simulink model "ModelMedusa"  (R2022b)
settings: Solver=FixedStepDiscrete  StartTime=0.0  StopTime=1  RelTol=1e-3  EnableMultiTasking=on
InitFcn:
  | % Initialize model
  | run(['ModelInit.m']);
  | 
  | % load library data
  | GainLibrary_data;
StartFcn:
  | % make sure all the simulated RTC requests are found
  | %RTC_SIM_OBJ.ValidateREQs();
model workspace (MAT data in the model file):
  PreampVolumeTable_Idx = Simulink.Signal
  PreampVolumeTable_Idx.DataType = 'auto'
  PreampVolumeTable_Idx.Dimensions = -1
  PreampVolumeTable_Idx.DimensionsMode = 'auto'
  PreampVolumeTable_Idx.Complexity = 'auto'
  PreampVolumeTable_Idx.SampleTime = -1
  PreampVolumeTable_Idx.SamplingMode = 'auto'
  PreampVolumeTable_Idx.InitialValue = 'uint8([0 255 255 255 255 255])'
  Range = Simulink.Signal
  Range.DataType = 'auto'
  Range.Dimensions = -1
  Range.DimensionsMode = 'auto'
  Range.Complexity = 'auto'
  Range.SampleTime = -1
  Range.SamplingMode = 'auto'
  Table_Idx = Simulink.Signal
  Table_Idx.DataType = 'auto'
  Table_Idx.Dimensions = -1
  Table_Idx.DimensionsMode = 'auto'
  Table_Idx.Complexity = 'auto'
  Table_Idx.SampleTime = -1
  Table_Idx.SamplingMode = 'auto'
undefined symbols (not defined in the file): Config, IFIR, Ifir, MedusaConfig, numAudioIn, Row, sys_defs, VLSConfig
libraries: TuneVar x16, FeaturePath x15, MedusaDelays x9, RTC x5, TOP x5, SampleRateConverter x4, dspindex x3, EdgePorts x2, MedusaCaeEnable x2, FIREven x2, VLSGains x2, dspsrcs4 x2
(part 1 of 2)
settings Model: Creator=kl13806  LastModifiedBy=sc48041
settings SolverCC: AlgebraicLoopSolver=TrustRegion  AutoInsertRateTranBlk=on
settings OptimizationCC: DefaultParameterBehavior=Inlined  DefaultUnderspecifiedDataType=single  ZeroExternalMemoryAtStartup=off  ZeroInternalMemoryAtStartup=off  MaxStackSize=2048  DifferentSizesBufferReuse=on  EfficientTunableParamExpr=on
settings DebuggingCC: InheritedTsInSrcMsg=none  MultiTaskDSMMsg=none  MultiTaskRateTransMsg=warning  ParameterPrecisionLossMsg=none  ParameterTunabilityLossMsg=error  UnconnectedInputMsg=warning  UnconnectedOutputMsg=warning  UnconnectedLineMsg=warning  BusObjectLabelMismatch=none  UnknownTsInhSupMsg=none  SFUnexpectedBacktrackingDiag=warning  SFNoUnconditionalDefaultTransitionDiag=warning  SFExecutionAtInitializationDiag=none  SFMachineParentedDataDiag=warning  ArithmeticOperatorsInVariantConditions=warning
settings HardwareCC: ProdBitPerDouble=32  ProdBitPerPointer=32  ProdBitPerSizeT=32  ProdBitPerPtrDiffT=32  ProdLargestAtomicInteger=Long  ProdLargestAtomicFloat=Double  ProdWordSize=32  ProdHWDeviceType=Qualcomm->Hexagon  TargetBitPerPointer=64  TargetBitPerSizeT=64  TargetBitPerPtrDiffT=64  TargetLargestAtomicInteger=Integer  TargetLongLongMode=on  TargetIntDivRoundTo=Zero  TargetEndianess=LittleEndian  TargetWordSize=64  TargetHWDeviceType=MATLAB Host  ProdEqTarget=off
settings ModelReferenceCC: EnableRefExpFcnMdlSchedulingChecks=on
settings SFSimCC: SimUseLocalCustomCode=off  MATLABDynamicMemAlloc=off  CustomCodeUndefinedFunction=UseInterfaceOnly
settings RTWCC: Description=Embedded Coder (host-based shared library target)  SystemTargetFile=ert_shrlib.tlc  GenCodeOnly=on  TemplateMakefile=ert_default_tmf  GenerateReport=on  RetainRTWFile=on  RTWUseLocalCustomCode=off  BuildConfiguration=Faster Runs  IncludeHyperlinkInReport=on  LaunchReport=on  GenerateTraceInfo=on  GenerateTraceReport=on  GenerateTraceReportSl=on  GenerateTraceReportSf=on  GenerateTraceReportEml=on  GenerateCodeMetricsReport=on  GenerateCodeReplacementReport=on
settings CodeAppCC: ForceParamTrailComments=on  IgnoreCustomStorageClasses=off  MaxIdLength=61  OperatorAnnotations=on  SimulinkDataObjDesc=on  SFDataObjDesc=on  MATLABFcnDesc=on  InsertBlockDesc=on  StateflowObjectComments=on  MATLABSourceComments=on
settings STFCustomTargetCC: TargetLangStandard=C99 (ISO)  CodeReplacementLibrary=Qualcomm Hexagon DSP code replacement library  ParMdlRefBuildCompliant=on  CompOptLevelCompliant=on  CombineOutputUpdateFcns=on  ERTCustomFileBanners=on  SupportNonFinite=off  SupportContinuousTime=off  SupportNonInlinedSFcns=off  RemoveResetFunc=on  SupportVariableSizeSignals=on  MATLABClassNameForMDSCustomization=Simulink.SoftwareTarget.ERTCustomization  ModelStepFunctionPrototypeControlCompliant=on  UseToolchainInfoCompliant=on  SystemTargetFile=ert_shrlib.tlc
settings ERTTargetCC: TargetLangStandard=C99 (ISO)  CodeReplacementLibrary=Qualcomm Hexagon DSP code replacement library  MultiwordLength=2048  ConcurrentExecutionCompliant=off  SupportNonFinite=off  SupportVariableSizeSignals=on  CPPClassGenCompliant=off  InlinedParameterPlacement=NonHierarchical  ERTCustomFileTemplate=example_file_process.tlc  IndentStyle=Allman  IndentSize=4
settings ConfigComp: CovMetricSettings=dw  CovSaveCumulativeToWorkspaceVar=on  CovSaveSingleToWorkspaceVar=on  CovExternalEMLEnable=off

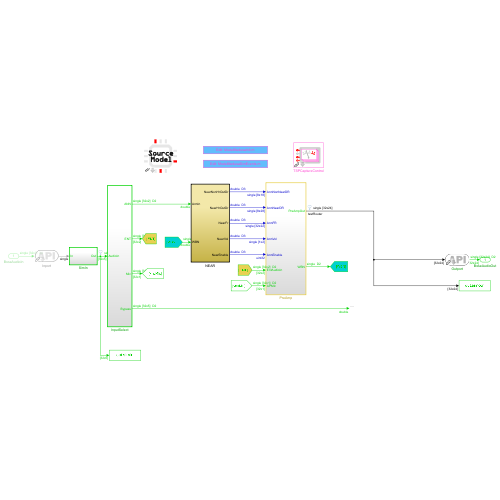
[thumbnail: Simulink's stored preview of the top-level diagram]
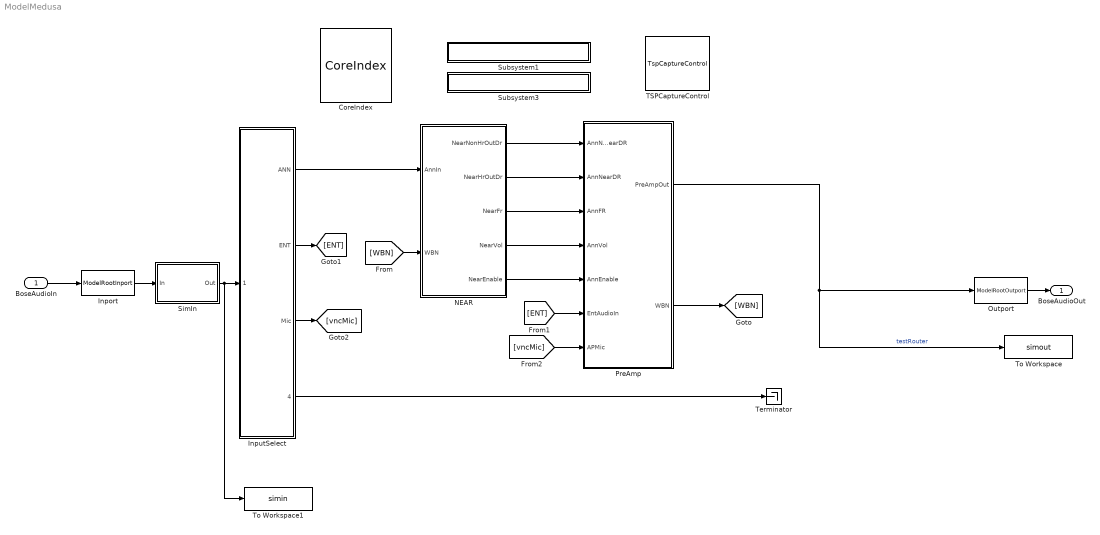
== system ModelMedusa ==
  BoseAudioIn : Inport  OutDataTypeStr=single  PortDimensions=[sys_defs.frameSize numAudioIn]  SampleTime=1/sys_defs.Fs * sys_defs.frameSize
  CoreIndex : FeaturePath/CoreIndex  Role=Source Model  CoreIndex=8  Config=[]  AddressingMode=Directly include core number in message identifiers (i.e. simple and static)  CrossCoreApi=None  CrossCoreAllocation=None  CrossCoreSampleTime=-1  BasePeriod=[]  TriggerInit=[-15 -776 80 -679]
      settings: SourceProductName=Bose Talaria
  Inport : EdgePorts/ModelRootInport  Config=ModelRootIn
      settings: SourceProductName=Bose Talaria
  InputSelect : Subsystem  TreatAsAtomicUnit=on
      settings: RTWSystemCode=Nonreusable function
  NEAR : Subsystem  TreatAsAtomicUnit=on
  Outport : EdgePorts/ModelRootOutport  Config=ModelRootOut
      settings: SourceProductName=Bose Talaria
  PreAmp : Subsystem  TreatAsAtomicUnit=on
  SimIn : Subsystem  TreatAsAtomicUnit=on
  Subsystem1 : Subsystem  mask{filename=Init.m}
      settings: OpenFcn=edit([ ModelRootName() get(gcbh,'filename') ]);
      mask Display: disp(['Edit: ' ModelRootName() get(gcbh,'filename')]);
  Subsystem3 : Subsystem  mask{filename=SimEvents.m}
      settings: OpenFcn=edit([ ModelRootName() get(gcbh,'filename') ]);
      mask Display: disp(['Edit: ' ModelRootName() get(gcbh,'filename')]);
  TSPCaptureControl : TSP/TspCaptureControl  TriggerInit=[415 -766 500 -694]
      settings: SourceProductName=Bose Talaria
  Terminator : Terminator
  To Workspace : ToWorkspace  VariableName=simout  SaveFormat=Timeseries  SampleTime=-1
  To Workspace1 : ToWorkspace  VariableName=simin  SaveFormat=Timeseries  SampleTime=-1
  BoseAudioOut : Outport  VectorParamsAs1DForOutWhenUnconnected=off
  wires:
  SimIn/1(Out) -> To Workspace1/1, InputSelect/1(AudioIn)
  BoseAudioIn/1 -> Inport/1
  Inport/1 -> SimIn/1(In)
  Outport/1 -> BoseAudioOut/1
  InputSelect/1(ANN) -> NEAR/1(AnnIn)
  [WBN] -> NEAR/2(WBN)
  NEAR/5(NearEnable) -> PreAmp/5(AnnEnable)
  NEAR/4(NearVol) -> PreAmp/4(AnnVol)
  NEAR/3(NearFr) -> PreAmp/3(AnnFR)
  PreAmp/2(WBN) -> [WBN]
  NEAR/1(NearNonHrOutDr) -> PreAmp/1(AnnNonNearDR)
  NEAR/2(NearHrOutDr) -> PreAmp/2(AnnNearDR)
  InputSelect/2(ENT) -> [ENT]
  [ENT] -> PreAmp/6(EntAudioIn)
  InputSelect/3(Mic) -> [vncMic]
  [vncMic] -> PreAmp/7(APMic)
  InputSelect/4(Bypass) -> Terminator/1
  PreAmp/1(PreAmpOut) -> To Workspace/1, Outport/1  "testRouter"

== system ModelMedusa/InputSelect ==
  AudioIn : Inport
  FeaturePath : FeaturePath/FeaturePath  FeatureName=InputSelect  IsGroup=on  GroupNumber=0  IsModule=on  TriggerInit=[105 216 220 329]
      settings: SourceProductName=Bose Talaria
  Partition : FeaturePath/Partition  PartitionNumber=0  TriggerInit=[250 241 295 309]
      settings: SourceProductName=Bose Talaria
  Reset : Subsystem  Commented=on
  Variable Selector1 : dspindex/Variable Selector  NumInputs=1  rowsOrCols=Columns  IdxMode=Fixed  Elements=entMap  ZerOneIdxMode=One-based  errmode=Clip Index  FillMode=on  FillValues=0
  Variable Selector2 : dspindex/Variable Selector  NumInputs=1  rowsOrCols=Columns  IdxMode=Fixed  Elements=annMap  ZerOneIdxMode=One-based  errmode=Clip Index  FillMode=on  FillValues=0
  Variable Selector3 : dspindex/Variable Selector  NumInputs=1  rowsOrCols=Columns  IdxMode=Fixed  Elements=vncMic  ZerOneIdxMode=One-based  errmode=Clip Index  FillMode=on  FillValues=0
  router : Router/Router  nInRouterMask=inputSelectChanIn  nOutRouterMask=inputSelectChanOut  outputMapDefaultRouterMask=inputSelectOutputMap
  ANN : Outport
  ENT : Outport  Port=2  VectorParamsAs1DForOutWhenUnconnected=off
  Mic : Outport  Port=3
  Bypass : Outport  Port=4  VectorParamsAs1DForOutWhenUnconnected=off
  wires:
  Variable Selector1/1 -> ENT/1
  AudioIn/1 -> Bypass/1, router/1
  router/1 -> Variable Selector3/1, Variable Selector2/1, Variable Selector1/1
  Variable Selector2/1 -> ANN/1
  Variable Selector3/1 -> Mic/1

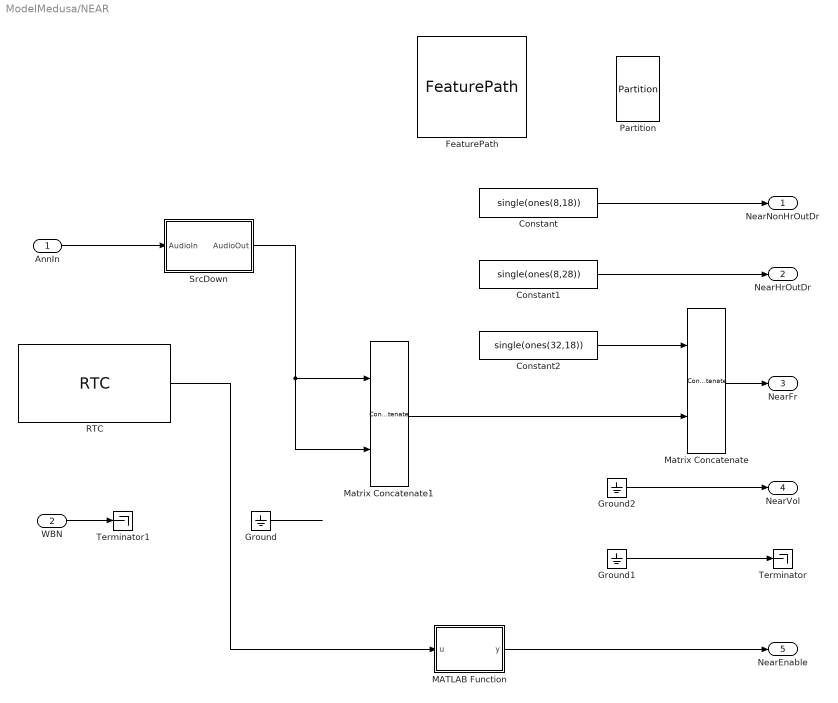
== system ModelMedusa/NEAR ==
  AnnIn : Inport
  WBN : Inport  Port=2
  Constant : Constant  Value=single(ones(8,18))
  Constant1 : Constant  Value=single(ones(8,28))
  Constant2 : Constant  Value=single(ones(32,18))
  FeaturePath : FeaturePath/FeaturePath  FeatureName=Near  IsGroup=on  GroupNumber=1  IsModule=on  TriggerInit=[15 -306 130 -199]
      settings: SourceProductName=Bose Talaria
  Ground : Ground
  Ground1 : Ground
  Ground2 : Ground
  MATLAB Function : MATLAB Function  TreatAsAtomicUnit=on
  Matrix Concatenate : Concatenate  Mode=Multidimensional array  ConcatenateDimension=2
  Matrix Concatenate1 : Concatenate  Mode=Multidimensional array  ConcatenateDimension=2
  Partition : FeaturePath/Partition  PartitionNumber=0  TriggerInit=[225 -284 270 -216]
      settings: SourceProductName=Bose Talaria
  RTC : RTC/RTC  REQ_Priority=RTC_Mask.NormalPriority  RequestAtInit=off  EnableRequest=off  REQElemName1=Enable  REQElemType1=uint32  REQElemWidth1=1  REQElemInitial1=[0]  REQElemType2=uint32  REQElemWidth2=1  REQElemInitial2=[]  REQElemType3=uint32  REQElemWidth3=1  REQElemInitial3=[]  REQElemType4=uint32  REQElemWidth4=1  REQElemInitial4=[]  REQElemType5=uint32  REQElemWidth5=1  REQElemInitial5=[]  REQElemType6=uint32  REQElemWidth6=1  REQElemInitial6=[]  REQElemType7=uint32  REQElemWidth7=1  REQElemInitial7=[]  REQElemType8=uint32  REQElemWidth8=1  REQElemInitial8=[]  REQElemType9=uint32  REQElemWidth9=1  REQElemInitial9=[]  REQElemType10=uint32  REQElemWidth10=1  REQElemInitial10=[]  EnableResponse=on  EnableRSP_StatusIn=off  RSPElemType1=uint32  RSPElemWidth1=1  RSPElemType2=uint32  RSPElemWidth2=1  RSPElemType3=uint32  RSPElemWidth3=1  RSPElemType4=uint32  RSPElemWidth4=1  RSPElemType5=uint32  RSPElemWidth5=1  RSPElemType6=uint32  RSPElemWidth6=1  RSPElemType7=uint32  RSPElemWidth7=1  RSPElemType8=uint32  RSPElemWidth8=1  RSPElemType9=uint32  RSPElemWidth9=1  RSPElemType10=uint32  RSPElemWidth10=1  EnableNotification=off  EnableNTF_PrepTrig=off  NTFElemType1=uint32  NTFElemWidth1=1  NTFElemType2=uint32  NTFElemWidth2=1  NTFElemType3=uint32  NTFElemWidth3=1  NTFElemType4=uint32  NTFElemWidth4=1  NTFElemType5=uint32  NTFElemWidth5=1  NTFElemType6=uint32  NTFElemWidth6=1  NTFElemType7=uint32  NTFElemWidth7=1  NTFElemType8=uint32  NTFElemWidth8=1  NTFElemType9=uint32  NTFElemWidth9=1  NTFElemType10=uint32  NTFElemWidth10=1  MaskMessageName=Enable
      settings: SourceProductName=Bose Talaria
  SrcDown : Subsystem  TreatAsAtomicUnit=on
      settings: RTWSystemCode=Nonreusable function
  Terminator : Terminator
  Terminator1 : Terminator
  NearNonHrOutDr : Outport
  NearHrOutDr : Outport  Port=2
  NearFr : Outport  Port=3
  NearVol : Outport  Port=4
  NearEnable : Outport  Port=5
  wires:
  Constant/1 -> NearNonHrOutDr/1
  AnnIn/1 -> SrcDown/1(AudioIn)
  Constant1/1 -> NearHrOutDr/1
  Constant2/1 -> Matrix Concatenate/1
  Matrix Concatenate1/1 -> Matrix Concatenate/2
  Matrix Concatenate/1 -> NearFr/1
  Ground2/1 -> NearVol/1
  Ground1/1 -> Terminator/1
  RTC/1 -> MATLAB Function/1(u)
  MATLAB Function/1(y) -> NearEnable/1
  SrcDown/1(AudioOut) -> Matrix Concatenate1/2, Matrix Concatenate1/1
  Ground/1 -> ?
  WBN/1 -> Terminator1/1

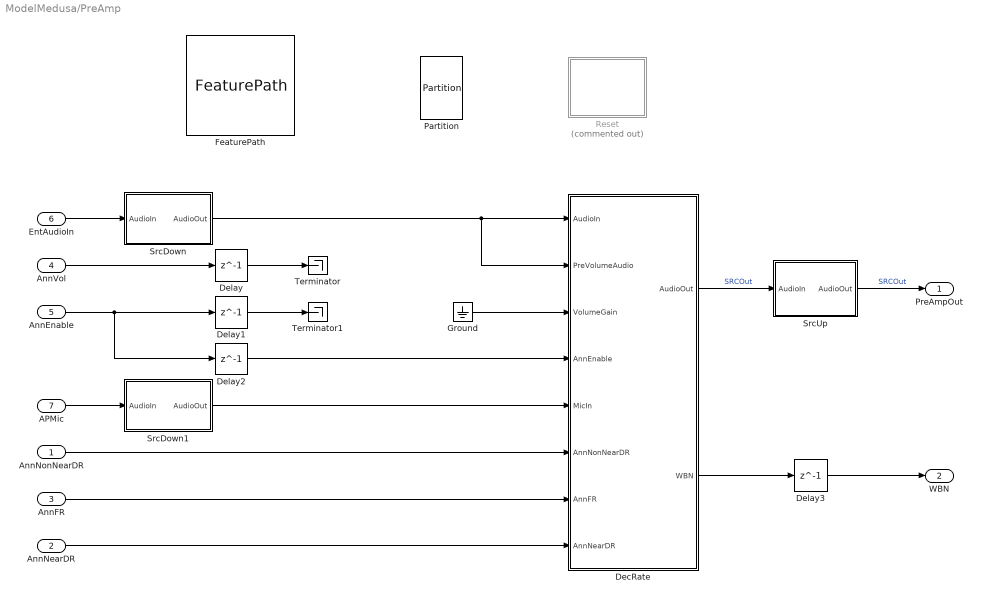
== system ModelMedusa/PreAmp ==
  AnnNonNearDR : Inport
  AnnNearDR : Inport  Port=2
  AnnFR : Inport  Port=3
  AnnVol : Inport  Port=4
  AnnEnable : Inport  Port=5
  EntAudioIn : Inport  Port=6
  APMic : Inport  Port=7
  DecRate : Subsystem
  Delay{,1..3} (4 alike) : Delay  DelayLength=1
  FeaturePath : FeaturePath/FeaturePath  FeatureName=PreAmp  IsGroup=on  GroupNumber=2  IsModule=on  TriggerInit=[-135 -246 -20 -139]
      settings: SourceProductName=Bose Talaria
  Ground : Ground
  Partition : FeaturePath/Partition  PartitionNumber=0  TriggerInit=[115 -224 160 -156]
      settings: SourceProductName=Bose Talaria
  Reset : Subsystem  Commented=on
  SrcDown : Subsystem  TreatAsAtomicUnit=on
      settings: RTWSystemCode=Nonreusable function
  SrcDown1 : Subsystem  TreatAsAtomicUnit=on
      settings: RTWSystemCode=Nonreusable function
  SrcUp : Subsystem  TreatAsAtomicUnit=on
      settings: RTWSystemCode=Nonreusable function
  Terminator : Terminator
  Terminator1 : Terminator
  PreAmpOut : Outport  VectorParamsAs1DForOutWhenUnconnected=off
  WBN : Outport  Port=2
  wires:
  EntAudioIn/1 -> SrcDown/1(AudioIn)
  DecRate/1(AudioOut) -> SrcUp/1(AudioIn)  "SRCOut"
  SrcUp/1(AudioOut) -> PreAmpOut/1  "SRCOut"
  Delay3/1 -> WBN/1
  AnnVol/1 -> Delay/1
  AnnEnable/1 -> Delay2/1, Delay1/1
  Delay/1 -> Terminator/1
  Delay1/1 -> Terminator1/1
  AnnNonNearDR/1 -> DecRate/6(AnnNonNearDR)
  AnnNearDR/1 -> DecRate/8(AnnNearDR)
  AnnFR/1 -> DecRate/7(AnnFR)
  APMic/1 -> SrcDown1/1(AudioIn)
  SrcDown/1(AudioOut) -> DecRate/2(PreVolumeAudio), DecRate/1(AudioIn)
  Ground/1 -> DecRate/3(VolumeGain)
  Delay2/1 -> DecRate/4(AnnEnable)
  DecRate/2(WBN) -> Delay3/1
  SrcDown1/1(AudioOut) -> DecRate/5(MicIn)

== system ModelMedusa/SimIn ==
  In : Inport  OutDataTypeStr=single  SampleTime=1/sys_defs.Fs * sys_defs.frameSize
  Colored Noise : dspsrcs4/Colored Noise  Commented=on  Color=pink  InverseFrequencyPower=1  BoundedOutput=on  NumChannels=2  OutputDataType=single  SamplesPerFrame=32  SampleTime=1/48000  RandomStream=mt19937ar with seed  Seed=67  SimulateUsing=Interpreted execution
  Sine Wave : dspsrcs4/Sine Wave  Amplitude=[0.1*ones(1,numAudioIn)]  Frequency=[150 225 200 275 325]  Phase=zeros(1,numAudioIn)  SampleMode=Discrete  OutComplex=Real  CompMethod=Trigonometric fcn  TableSize=Speed  SampleTime=1/sys_defs.Fs  SamplesPerFrame=sys_defs.frameSize  ResetState=Restart at time zero  OutputFrames=off  dataType=single  wordLen=16  udDataType=sfix(16)  fracBitsMode=Best precision  numFracBits=15  OutDataTypeStr=single  LastOutDataTypeStr=single
  Variant Source : VariantSource  VariantControlMode=sim codegen switching  ShowConditionOnBlock=on
  Out : Outport  VectorParamsAs1DForOutWhenUnconnected=off
  wires:
  In/1 -> Variant Source/2
  Variant Source/1 -> Out/1
  Sine Wave/1 -> Variant Source/1

== system ModelMedusa/Subsystem1 ==

== system ModelMedusa/Subsystem3 ==

== system ModelMedusa/InputSelect/Reset ==
  MATLAB Function : MATLAB Function  TreatAsAtomicUnit=on
  RTC : RTC/RTC  REQ_Priority=RTC_Mask.NormalPriority  RequestAtInit=off  EnableRequest=on  REQElemType1=uint32  REQElemWidth1=1  REQElemInitial1=[]  REQElemType2=uint32  REQElemWidth2=1  REQElemInitial2=[]  REQElemType3=uint32  REQElemWidth3=1  REQElemInitial3=[]  REQElemType4=uint32  REQElemWidth4=1  REQElemInitial4=[]  REQElemType5=uint32  REQElemWidth5=1  REQElemInitial5=[]  REQElemType6=uint32  REQElemWidth6=1  REQElemInitial6=[]  REQElemType7=uint32  REQElemWidth7=1  REQElemInitial7=[]  REQElemType8=uint32  REQElemWidth8=1  REQElemInitial8=[]  REQElemType9=uint32  REQElemWidth9=1  REQElemInitial9=[]  REQElemType10=uint32  REQElemWidth10=1  REQElemInitial10=[]  EnableResponse=on  EnableRSP_StatusIn=off  RSPElemType1=uint32  RSPElemWidth1=1  RSPElemType2=uint32  RSPElemWidth2=1  RSPElemType3=uint32  RSPElemWidth3=1  RSPElemType4=uint32  RSPElemWidth4=1  RSPElemType5=uint32  RSPElemWidth5=1  RSPElemType6=uint32  RSPElemWidth6=1  RSPElemType7=uint32  RSPElemWidth7=1  RSPElemType8=uint32  RSPElemWidth8=1  RSPElemType9=uint32  RSPElemWidth9=1  RSPElemType10=uint32  RSPElemWidth10=1  EnableNotification=off  EnableNTF_PrepTrig=off  NTFElemType1=uint32  NTFElemWidth1=1  NTFElemType2=uint32  NTFElemWidth2=1  NTFElemType3=uint32  NTFElemWidth3=1  NTFElemType4=uint32  NTFElemWidth4=1  NTFElemType5=uint32  NTFElemWidth5=1  NTFElemType6=uint32  NTFElemWidth6=1  NTFElemType7=uint32  NTFElemWidth7=1  NTFElemType8=uint32  NTFElemWidth8=1  NTFElemType9=uint32  NTFElemWidth9=1  NTFElemType10=uint32  NTFElemWidth10=1  MaskMessageName=Reset
      settings: SourceProductName=Bose Talaria
  wires:
  RTC/1 -> MATLAB Function/Trigger

== system ModelMedusa/NEAR/SrcDown ==
  AudioIn : Inport
  Frame Conversion1 : FrameConversion  OutFrame=Sample-based
  Frame Conversion2 : FrameConversion
  SampleRateConverter : SampleRateConverter/SampleRateConverter  UPFACTOR=12  DOWNFACTOR=13  OUTFRAME_SIZE=-1  RATE_SELECTOR=Input Sample Rate  FS=48000  FPASSBAND=16500  FHEARING=19000  PASSBAND_RIPPLE=60  STOPBAND_ATTENUATION=60
  AudioOut : Outport
  wires:
  SampleRateConverter/1 -> Frame Conversion1/1
  AudioIn/1 -> Frame Conversion2/1
  Frame Conversion1/1 -> AudioOut/1
  Frame Conversion2/1 -> SampleRateConverter/1

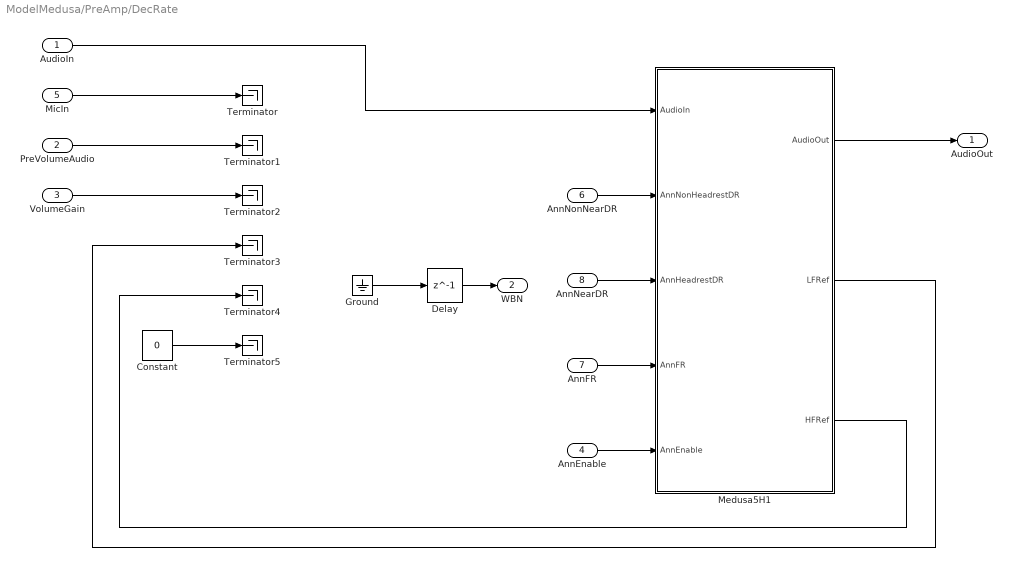
== system ModelMedusa/PreAmp/DecRate ==
  AudioIn : Inport
  PreVolumeAudio : Inport  Port=2
  VolumeGain : Inport  Port=3
  AnnEnable : Inport  Port=4
  MicIn : Inport  Port=5
  AnnNonNearDR : Inport  Port=6
  AnnFR : Inport  Port=7
  AnnNearDR : Inport  Port=8
  Constant : Constant  Value=0
  Delay : Delay  DelayLength=1
  Ground : Ground
  Medusa5H1 : Subsystem
  Terminator{,1..5} (6 alike) : Terminator
  AudioOut : Outport
  WBN : Outport  Port=2
  wires:
  Medusa5H1/1(AudioOut) -> AudioOut/1
  PreVolumeAudio/1 -> Terminator1/1
  MicIn/1 -> Terminator/1
  Ground/1 -> Delay/1
  Delay/1 -> WBN/1
  VolumeGain/1 -> Terminator2/1
  Medusa5H1/2(LFRef) -> Terminator3/1
  Medusa5H1/3(HFRef) -> Terminator4/1
  Constant/1 -> Terminator5/1
  AnnEnable/1 -> Medusa5H1/5(AnnEnable)
  AnnNonNearDR/1 -> Medusa5H1/2(AnnNonHeadrestDR)
  AnnNearDR/1 -> Medusa5H1/3(AnnHeadrestDR)
  AnnFR/1 -> Medusa5H1/4(AnnFR)
  AudioIn/1 -> Medusa5H1/1(AudioIn)

== system ModelMedusa/PreAmp/Reset ==
  MATLAB Function : MATLAB Function  TreatAsAtomicUnit=on
  RTC : RTC/RTC  REQ_Priority=RTC_Mask.NormalPriority  RequestAtInit=off  EnableRequest=on  REQElemType1=uint32  REQElemWidth1=1  REQElemInitial1=[]  REQElemType2=uint32  REQElemWidth2=1  REQElemInitial2=[]  REQElemType3=uint32  REQElemWidth3=1  REQElemInitial3=[]  REQElemType4=uint32  REQElemWidth4=1  REQElemInitial4=[]  REQElemType5=uint32  REQElemWidth5=1  REQElemInitial5=[]  REQElemType6=uint32  REQElemWidth6=1  REQElemInitial6=[]  REQElemType7=uint32  REQElemWidth7=1  REQElemInitial7=[]  REQElemType8=uint32  REQElemWidth8=1  REQElemInitial8=[]  REQElemType9=uint32  REQElemWidth9=1  REQElemInitial9=[]  REQElemType10=uint32  REQElemWidth10=1  REQElemInitial10=[]  EnableResponse=on  EnableRSP_StatusIn=off  RSPElemType1=uint32  RSPElemWidth1=1  RSPElemType2=uint32  RSPElemWidth2=1  RSPElemType3=uint32  RSPElemWidth3=1  RSPElemType4=uint32  RSPElemWidth4=1  RSPElemType5=uint32  RSPElemWidth5=1  RSPElemType6=uint32  RSPElemWidth6=1  RSPElemType7=uint32  RSPElemWidth7=1  RSPElemType8=uint32  RSPElemWidth8=1  RSPElemType9=uint32  RSPElemWidth9=1  RSPElemType10=uint32  RSPElemWidth10=1  EnableNotification=off  EnableNTF_PrepTrig=off  NTFElemType1=uint32  NTFElemWidth1=1  NTFElemType2=uint32  NTFElemWidth2=1  NTFElemType3=uint32  NTFElemWidth3=1  NTFElemType4=uint32  NTFElemWidth4=1  NTFElemType5=uint32  NTFElemWidth5=1  NTFElemType6=uint32  NTFElemWidth6=1  NTFElemType7=uint32  NTFElemWidth7=1  NTFElemType8=uint32  NTFElemWidth8=1  NTFElemType9=uint32  NTFElemWidth9=1  NTFElemType10=uint32  NTFElemWidth10=1  MaskMessageName=Reset
      settings: SourceProductName=Bose Talaria
  wires:
  RTC/1 -> MATLAB Function/Trigger

== system ModelMedusa/PreAmp/SrcDown ==
  AudioIn : Inport
  Frame Conversion1 : FrameConversion  OutFrame=Sample-based
  Frame Conversion2 : FrameConversion
  SampleRateConverter : SampleRateConverter/SampleRateConverter  UPFACTOR=12  DOWNFACTOR=13  OUTFRAME_SIZE=-1  RATE_SELECTOR=Input Sample Rate  FS=48000  FPASSBAND=16500  FHEARING=19000  PASSBAND_RIPPLE=60  STOPBAND_ATTENUATION=60
  AudioOut : Outport
  wires:
  SampleRateConverter/1 -> Frame Conversion1/1
  AudioIn/1 -> Frame Conversion2/1
  Frame Conversion1/1 -> AudioOut/1
  Frame Conversion2/1 -> SampleRateConverter/1

== system ModelMedusa/PreAmp/SrcDown1 ==
  AudioIn : Inport
  Frame Conversion1 : FrameConversion  OutFrame=Sample-based
  Frame Conversion2 : FrameConversion
  SampleRateConverter : SampleRateConverter/SampleRateConverter  UPFACTOR=12  DOWNFACTOR=13  OUTFRAME_SIZE=-1  RATE_SELECTOR=Input Sample Rate  FS=48000  FPASSBAND=16500  FHEARING=19000  PASSBAND_RIPPLE=60  STOPBAND_ATTENUATION=60
  AudioOut : Outport
  wires:
  SampleRateConverter/1 -> Frame Conversion1/1
  AudioIn/1 -> Frame Conversion2/1
  Frame Conversion1/1 -> AudioOut/1
  Frame Conversion2/1 -> SampleRateConverter/1

== system ModelMedusa/PreAmp/SrcUp ==
  AudioIn : Inport
  Frame Conversion : FrameConversion
  Frame Conversion1 : FrameConversion  OutFrame=Sample-based
  SampleRateConverter1 : SampleRateConverter/SampleRateConverter  UPFACTOR=13  DOWNFACTOR=12  OUTFRAME_SIZE=-1  RATE_SELECTOR=Input Sample Rate  FS=48000  FPASSBAND=16500  FHEARING=19000  PASSBAND_RIPPLE=60  STOPBAND_ATTENUATION=60
  AudioOut : Outport
  wires:
  SampleRateConverter1/1 -> Frame Conversion1/1
  Frame Conversion/1 -> SampleRateConverter1/1
  Frame Conversion1/1 -> AudioOut/1
  AudioIn/1 -> Frame Conversion/1

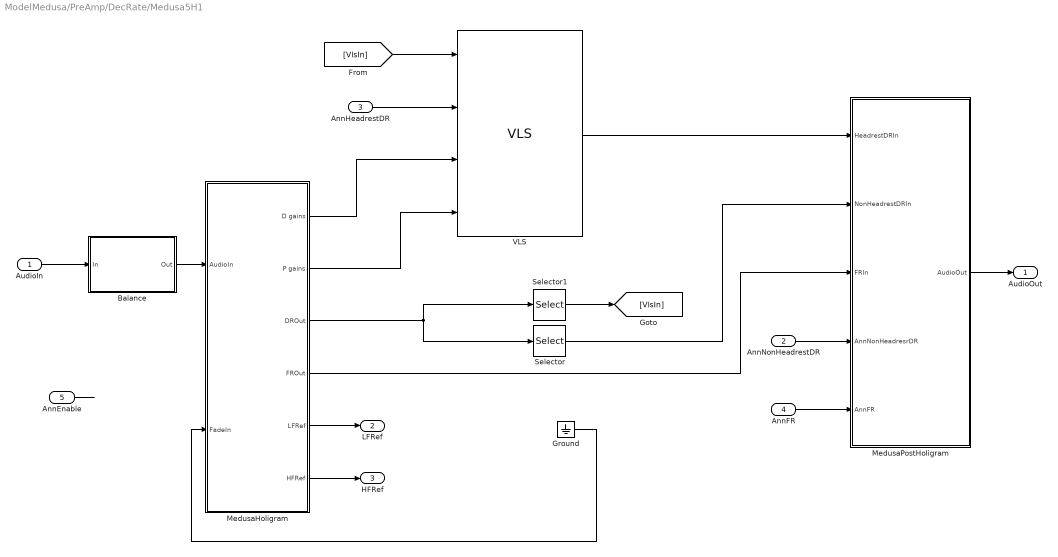
== system ModelMedusa/PreAmp/DecRate/Medusa5H1 ==
  AudioIn : Inport
  AnnNonHeadrestDR : Inport  Port=2
  AnnHeadrestDR : Inport  Port=3
  AnnFR : Inport  Port=4
  AnnEnable : Inport  Port=5
  Balance : Subsystem
  Ground : Ground
  MedusaHoligram : Subsystem  AncestorBlock=medusa5h1_stereo/Medusa + Holigram  mask{config=MedusaConfig, vlsConfigStruct=VLSConfig}
      mask prompts: config "Medusa config struct name:"; vlsConfigStruct "VLS config struct name:"
      mask init:
      | tailCompEQ = config.tailCompEQ;
      | HRDelayConfig = vlsConfigStruct.HeadrestDelayConfig;
      settings: LibrarySourceBlock=medusa5h1_stereo/Medusa + Holigram
  MedusaPostHoligram : Subsystem
  Selector : Selector  NumberOfDimensions=2  InputPortWidth=3  IndexOptions=Select all,Index vector (dialog)  Indices=[1 3],1:18  OutputSizes=1,1
  Selector1 : Selector  NumberOfDimensions=2  InputPortWidth=3  IndexOptions=Select all,Index vector (dialog)  Indices=[1 3],19:30  OutputSizes=1,1
  VLS : VLS/VLS  configStruct=VLSConfig
  AudioOut : Outport
  LFRef : Outport  Port=2
  HFRef : Outport  Port=3
  wires:
  MedusaHoligram/6(HFRef) -> HFRef/1
  MedusaHoligram/2(P gains) -> VLS/4
  MedusaHoligram/1(D gains) -> VLS/3
  MedusaHoligram/5(LFRef) -> LFRef/1
  AudioIn/1 -> Balance/1(In)
  Balance/1(Out) -> MedusaHoligram/1(AudioIn)
  AnnEnable/1 -> ?
  AnnHeadrestDR/1 -> VLS/2
  MedusaHoligram/3(DROut) -> Selector/1, Selector1/1
  Selector1/1 -> [VlsIn]
  Ground/1 -> MedusaHoligram/2(FadeIn)
  AnnNonHeadrestDR/1 -> MedusaPostHoligram/4(AnnNonHeadresrDR)
  AnnFR/1 -> MedusaPostHoligram/5(AnnFR)
  VLS/1 -> MedusaPostHoligram/1(HeadrestDRIn)
  MedusaPostHoligram/1(AudioOut) -> AudioOut/1
  Selector/1 -> MedusaPostHoligram/2(NonHeadrestDRIn)
  MedusaHoligram/4(FROut) -> MedusaPostHoligram/3(FRIn)
  [VlsIn] -> VLS/1

== system ModelMedusa/PreAmp/DecRate/Medusa5H1/Balance ==
  In : Inport
  Balance : BalanceBtc/Balance  FeatureName=Balance  Config=Balance
      settings: SourceProductName=Bose Blocklib
  Out : Outport
  wires:
  Balance/1 -> Out/1
  In/1 -> Balance/1

== system ModelMedusa/PreAmp/DecRate/Medusa5H1/MedusaHoligram ==
  AudioIn : Inport
  FadeIn : Inport  Port=2  OutDataTypeStr=single
  FeaturePath : FeaturePath/FeaturePath  FeatureName=Medusa  IsGroup=off  GroupNumber=-1  IsModule=off  TriggerInit=[90 69 205 176]
      settings: SourceProductName=Bose Talaria
  Medusa5H1 Part 1 : Subsystem  TreatAsAtomicUnit=on
      settings: RTWSystemCode=Nonreusable function
  Medusa5H1 Part 2 : Subsystem  TreatAsAtomicUnit=on
      settings: RTWSystemCode=Nonreusable function
  Medusa5H1 Part 3 : Subsystem  TreatAsAtomicUnit=on
      settings: RTWSystemCode=Nonreusable function  FunctionWithSeparateData=on
  Medusa5H1 Part 4 : Subsystem  TreatAsAtomicUnit=on  RTWFcnName=MedusaHoligram  RTWFileName=MedusaHoligram
      settings: RTWSystemCode=Nonreusable function  RTWFcnNameOpts=User specified  RTWFileNameOpts=User specified  FunctionWithSeparateData=on
  Medusa5H1 Part 5 : Subsystem  TreatAsAtomicUnit=on
      settings: RTWSystemCode=Nonreusable function  FunctionWithSeparateData=on
  D gains : Outport
  P gains : Outport  Port=2
  DROut : Outport  Port=3
  FROut : Outport  Port=4
  LFRef : Outport  Port=5  VectorParamsAs1DForOutWhenUnconnected=off
  HFRef : Outport  Port=6  VectorParamsAs1DForOutWhenUnconnected=off
  wires:
  Medusa5H1 Part 1/4(CAEEnable) -> Medusa5H1 Part 2/4(CAEEnable)
  Medusa5H1 Part 2/3(HFRef) -> HFRef/1
  Medusa5H1 Part 5/2(FROut) -> FROut/1
  Medusa5H1 Part 5/1(DROut) -> DROut/1
  Medusa5H1 Part 4/2(FROut) -> Medusa5H1 Part 5/2(FRIn)
  Medusa5H1 Part 4/1(DROut) -> Medusa5H1 Part 5/1(DRIn)
  Medusa5H1 Part 3/1(D gains) -> D gains/1
  Medusa5H1 Part 3/3(HeadrestPremixOut) -> Medusa5H1 Part 4/1(HeadrestComps)
  Medusa5H1 Part 3/2(P gains) -> P gains/1
  Medusa5H1 Part 3/4(NonHeadrestPremixOut) -> Medusa5H1 Part 4/2(NonHeadrestComps)
  Medusa5H1 Part 1/1(LRbass) -> Medusa5H1 Part 3/1(Bass)
  [AudioIn] -> Medusa5H1 Part 2/1(AudioIn)
  Medusa5H1 Part 1/2(LRbp) -> Medusa5H1 Part 2/2(LRbp)
  Medusa5H1 Part 1/3(LRhp) -> Medusa5H1 Part 2/3(LRhp)
  Medusa5H1 Part 1/5(Mono) -> LFRef/1
  AudioIn/1 -> Medusa5H1 Part 1/1(AudioIn), [AudioIn]
  FadeIn/1 -> Medusa5H1 Part 3/4(FadeIn)
  Medusa5H1 Part 3/5(FRMixerOut) -> Medusa5H1 Part 4/3(FRSpkr)
  Medusa5H1 Part 2/1(DRComps) -> Medusa5H1 Part 3/2(DRComps)
  Medusa5H1 Part 2/2(FRComps) -> Medusa5H1 Part 3/3(FRComps)

== system ModelMedusa/PreAmp/DecRate/Medusa5H1/MedusaPostHoligram ==
  HeadrestDRIn : Inport
  NonHeadrestDRIn : Inport  Port=2
  FRIn : Inport  Port=3
  AnnNonHeadresrDR : Inport  Port=4
  AnnFR : Inport  Port=5
  Add : Sum
  Add1 : Sum
  MedusaPostHoligram : medusa5h1_stereo/Medusa Post Holigram  config=MedusaConfig
  AudioOut : Outport
  wires:
  HeadrestDRIn/1 -> MedusaPostHoligram/1
  MedusaPostHoligram/1 -> AudioOut/1
  NonHeadrestDRIn/1 -> Add/1
  AnnNonHeadresrDR/1 -> Add/2
  Add/1 -> MedusaPostHoligram/2
  FRIn/1 -> Add1/1
  Add1/1 -> MedusaPostHoligram/3
  AnnFR/1 -> Add1/2

== system ModelMedusa/PreAmp/DecRate/Medusa5H1/MedusaHoligram/Medusa5H1 Part 1 ==
  AudioIn : Inport
  Bass Manager Stereo : BassManager/MedusaBassManagerStereo  Config=Config.BassManager
  CAE Treble Boost : Subsystem  Variant=on
  Mean : dspstat3/Mean  run=off  InputProcessing=Columns as channels (frame based)  reset_popup=None  directionMode=Each row  dimension=1  roiEnable=off  roiType=Rectangles  roiPortion=Entire ROI  roiOutput=Individual statistics for each ROI  roiFlag=off  roundingMode=Floor  overflowMode=off  outputDataTypeStr=Inherit: Same as accumulator  outputMin=[]  outputMax=[]  outputLastDataTypeStr=Inherit: Same as accumulator
  Medusa Band Split Stereo : Subsystem  AncestorBlock=MedusaBandSplit/Medusa Band Split Stereo  mask(Medusa Band Split Stereo){configStruct=config.BandSplitConfig, numInputs=2}
      mask prompts: configStruct "Config struct name:"; numInputs "Number of inputs:"
      mask help:
      | This block performs bandsplitting and downsampling for stereo inputs used by Medusa system.
      |
      | Configuration struct needs to define the below fields with the exact names which are used inside the block.
      |
      | D: Decimation factor
      | ifir: Interpolated filter coefficients
      | fireven: Image rejection filter coefficients
      | upfir: Reconstruction filter coefficients
      | band_separation_delay: Alignment delay for the whole Bandsplit
      |
      | For more information and sample generation of config struct, please see 'Help'.
      settings: LibrarySourceBlock=MedusaBandSplit/Medusa Band Split Stereo
      mask Help:
      | Model that uses Band Split block need to call <i>MedusaBandSplitInit()</i> to generate <i>MedusaBandSplitConfig</i> in base workspace.
      | 
      | <b>Sample usage:</b>
      | 
      | MedusaConfig = generateMedusaConfig(auto_gen_sys_defs);
      | MedusaBandSplitInit(MedusaConfig);
      | or
      | DefaultMedusaConfig = generateMedusaConfig();
      | MedusaBandSplitInit(DefaultMedusaConfig);
  Partition : FeaturePath/Partition  PartitionNumber=2  TriggerInit=[375 -99 420 -31]
      settings: SourceProductName=Bose Talaria
  LRbass : Outport  VectorParamsAs1DForOutWhenUnconnected=off
  LRbp : Outport  Port=2  VectorParamsAs1DForOutWhenUnconnected=off
  LRhp : Outport  Port=3  VectorParamsAs1DForOutWhenUnconnected=off
  CAEEnable : Outport  Port=4
  Mono : Outport  Port=5  VectorParamsAs1DForOutWhenUnconnected=off
  wires:
  CAE Treble Boost/2(CAEEnable) -> CAEEnable/1
  AudioIn/1 -> CAE Treble Boost/1(AudioIn)  "L, R"
  Mean/1 -> Mono/1
  CAE Treble Boost/1(Out) -> Bass Manager Stereo/1, Mean/1  "L, R"
  Bass Manager Stereo/2 -> Medusa Band Split Stereo/1(LRhp)
  Medusa Band Split Stereo/1(LRbp) -> LRbp/1  "LRbp"
  Bass Manager Stereo/1 -> LRbass/1  "Lbass, Rbass"
  Medusa Band Split Stereo/2(LRtreble) -> LRhp/1  "LRtreble"

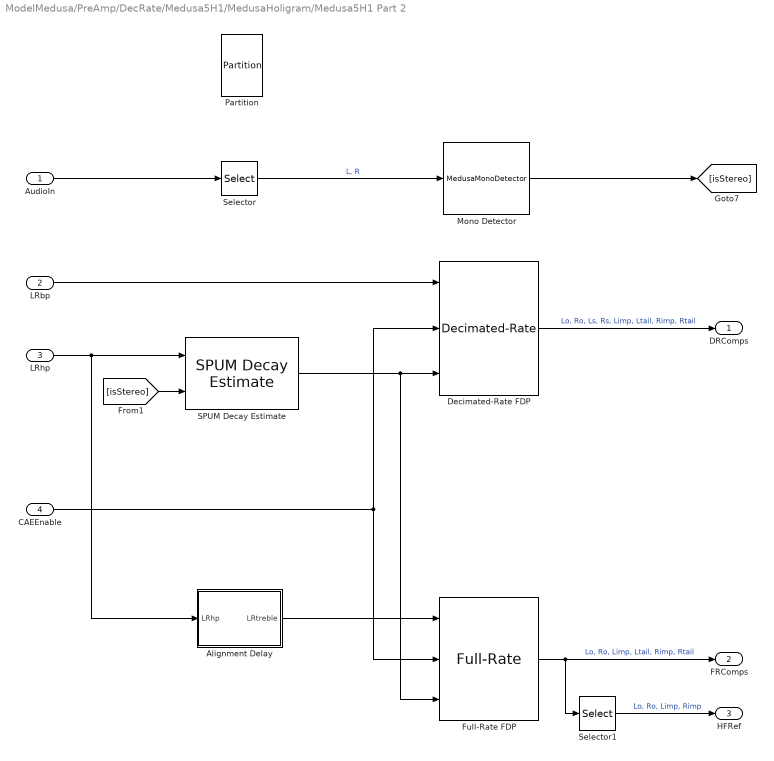
== system ModelMedusa/PreAmp/DecRate/Medusa5H1/MedusaHoligram/Medusa5H1 Part 2 ==
  AudioIn : Inport  OutDataTypeStr=single
  LRbp : Inport  Port=2
  LRhp : Inport  Port=3
  CAEEnable : Inport  Port=4
  Alignment Delay : Subsystem  TreatAsAtomicUnit=on
      settings: RTWSystemCode=Nonreusable function  FunctionWithSeparateData=on
  Decimated-Rate FDP : MedusaFDP/Decimated-Rate  FeatureName=DeciRate  configStruct=config.DRFDPConfig  RfftConfig=[]  RifftConfig=[]
  Full-Rate FDP : MedusaFullRateFDP/Full-Rate  FeatureName=FullRate  configStruct=config.FRFDPConfig  RfftConfig=[]  RifftConfig=[]
  Mono Detector : MonoDetector/MedusaMonoDetector  Config=Config.MonoDetector
  Partition : FeaturePath/Partition  PartitionNumber=3  TriggerInit=[825 236 870 304]
      settings: SourceProductName=Bose Talaria
  SPUM Decay Estimate : MedusaSPUMDecayEst/SPUM Decay Estimate  configStruct=config.FRFDPConfig
  Selector : Selector  NumberOfDimensions=2  InputPortWidth=3  IndexOptions=Select all,Index vector (dialog)  Indices=[1 3],[1,2]  OutputSizes=1,1
  Selector1 : Selector  NumberOfDimensions=2  InputPortWidth=3  IndexOptions=Select all,Index vector (dialog)  Indices=[1 3],[1 2 3 5]  OutputSizes=1,1
  DRComps : Outport  VectorParamsAs1DForOutWhenUnconnected=off
  FRComps : Outport  Port=2  VectorParamsAs1DForOutWhenUnconnected=off
  HFRef : Outport  Port=3
  wires:
  Alignment Delay/1(LRtreble) -> Full-Rate FDP/1
  CAEEnable/1 -> Full-Rate FDP/2, Decimated-Rate FDP/2
  Selector1/1 -> HFRef/1  "Lo, Ro, Limp, Rimp"
  Full-Rate FDP/1 -> FRComps/1, Selector1/1  "Lo, Ro, Limp, Ltail, Rimp, Rtail"
  [isStereo] -> SPUM Decay Estimate/2
  LRhp/1 -> SPUM Decay Estimate/1, Alignment Delay/1(LRhp)
  LRbp/1 -> Decimated-Rate FDP/1
  AudioIn/1 -> Selector/1
  Selector/1 -> Mono Detector/1  "L, R"
  Mono Detector/1 -> [isStereo]
  SPUM Decay Estimate/1 -> Decimated-Rate FDP/3, Full-Rate FDP/3
  Decimated-Rate FDP/1 -> DRComps/1  "Lo, Ro, Ls, Rs, Limp, Ltail, Rimp, Rtail"

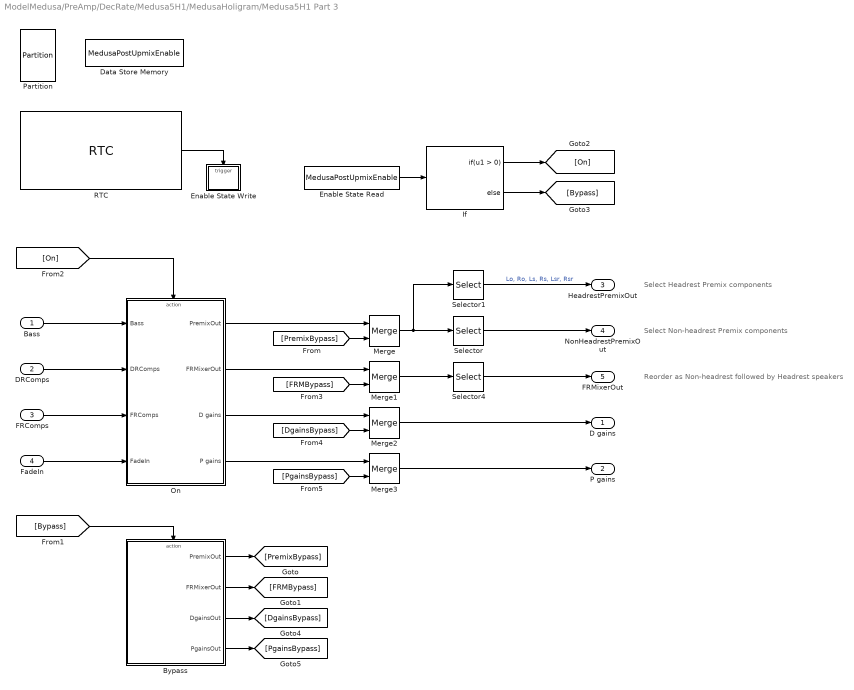
== system ModelMedusa/PreAmp/DecRate/Medusa5H1/MedusaHoligram/Medusa5H1 Part 3 ==
  note: Select Headrest Premix components
  note: Select Non-headrest Premix components
  note: Reorder as Non-headrest followed by Headrest speakers
  Bass : Inport
  DRComps : Inport  Port=2
  FRComps : Inport  Port=3
  FadeIn : Inport  Port=4
  Bypass : Subsystem
  Data Store Memory : DataStoreMemory  DataStoreName=MedusaPostUpmixEnable  ReadBeforeWriteMsg=warning  WriteAfterWriteMsg=warning  WriteAfterReadMsg=warning  InitialValue=1  ShowAdditionalParam=off  OutDataTypeStr=uint32
  Enable State Read : DataStoreRead  DataStoreName=MedusaPostUpmixEnable  IndexOptions=Index vector (dialog)  Indices=1  OutputSizes=1
  Enable State Write : Subsystem
  If : If
  Merge : Merge  InitialOutput=zeros(config.HoligramEQConfig.frameSize, config.PremixConfig.NumPremixOut)
  Merge1 : Merge  InitialOutput=Config.DefaultFullRateMixerOutput
  Merge2 : Merge  InitialOutput=zeros(config.numVLSGains, 1)
  Merge3 : Merge  InitialOutput=zeros(config.numVLSGains, 1)
  On : Subsystem
  Partition : FeaturePath/Partition  PartitionNumber=5  TriggerInit=[410 331 455 399]
      settings: SourceProductName=Bose Talaria
  RTC : RTC/RTC  REQ_Priority=RTC_Mask.NormalPriority  RequestAtInit=off  EnableRequest=on  REQElemType1=int32  REQElemWidth1=1  REQElemInitial1=[]  REQElemType2=uint32  REQElemWidth2=1  REQElemInitial2=[]  REQElemType3=uint32  REQElemWidth3=1  REQElemInitial3=[]  REQElemType4=uint32  REQElemWidth4=1  REQElemInitial4=[]  REQElemType5=uint32  REQElemWidth5=1  REQElemInitial5=[]  REQElemType6=uint32  REQElemWidth6=1  REQElemInitial6=[]  REQElemType7=uint32  REQElemWidth7=1  REQElemInitial7=[]  REQElemType8=uint32  REQElemWidth8=1  REQElemInitial8=[]  REQElemType9=uint32  REQElemWidth9=1  REQElemInitial9=[]  REQElemType10=uint32  REQElemWidth10=1  REQElemInitial10=[]  EnableResponse=on  EnableRSP_StatusIn=off  RSPElemType1=uint32  RSPElemWidth1=1  RSPElemType2=uint32  RSPElemWidth2=1  RSPElemType3=uint32  RSPElemWidth3=1  RSPElemType4=uint32  RSPElemWidth4=1  RSPElemType5=uint32  RSPElemWidth5=1  RSPElemType6=uint32  RSPElemWidth6=1  RSPElemType7=uint32  RSPElemWidth7=1  RSPElemType8=uint32  RSPElemWidth8=1  RSPElemType9=uint32  RSPElemWidth9=1  RSPElemType10=uint32  RSPElemWidth10=1  EnableNotification=off  EnableNTF_PrepTrig=off  NTFElemType1=uint32  NTFElemWidth1=1  NTFElemType2=uint32  NTFElemWidth2=1  NTFElemType3=uint32  NTFElemWidth3=1  NTFElemType4=uint32  NTFElemWidth4=1  NTFElemType5=uint32  NTFElemWidth5=1  NTFElemType6=uint32  NTFElemWidth6=1  NTFElemType7=uint32  NTFElemWidth7=1  NTFElemType8=uint32  NTFElemWidth8=1  NTFElemType9=uint32  NTFElemWidth9=1  NTFElemType10=uint32  NTFElemWidth10=1  MaskMessageName=PostUpmixDisable
      settings: SourceProductName=Bose Talaria
  Selector : Selector  NumberOfDimensions=2  InputPortWidth=3  IndexOptions=Select all,Index vector (dialog)  Indices=[1 3],config.NonHeadrestIdx  OutputSizes=1,1
  Selector1 : Selector  NumberOfDimensions=2  InputPortWidth=3  IndexOptions=Select all,Index vector (dialog)  Indices=[1 3],config.HeadrestIdx  OutputSizes=1,1
  Selector4 : Selector  NumberOfDimensions=2  InputPortWidth=3  IndexOptions=Select all,Index vector (dialog)  Indices=[1 3],config.FRMOutputIdx  OutputSizes=1,1
  D gains : Outport
  P gains : Outport  Port=2
  HeadrestPremixOut : Outport  Port=3  VectorParamsAs1DForOutWhenUnconnected=off
  NonHeadrestPremixOut : Outport  Port=4  VectorParamsAs1DForOutWhenUnconnected=off
  FRMixerOut : Outport  Port=5  VectorParamsAs1DForOutWhenUnconnected=off
  wires:
  Selector1/1 -> HeadrestPremixOut/1  "Lo, Ro, Ls, Rs, Lsr, Rsr"
  Selector/1 -> NonHeadrestPremixOut/1
  Merge3/1 -> P gains/1
  Merge2/1 -> D gains/1
  On/4(P gains) -> Merge3/1
  On/3(D gains) -> Merge2/1
  Merge1/1 -> Selector4/1
  On/2(FRMixerOut) -> Merge1/1
  RTC/1 -> Enable State Write/Trigger
  [On] -> On/Action
  Enable State Read/1 -> If/1
  If/2 -> [Bypass]
  If/1 -> [On]
  Merge/1 -> Selector/1, Selector1/1
  On/1(PremixOut) -> Merge/1
  [Bypass] -> Bypass/Action
  DRComps/1 -> On/2(DRComps)
  Bass/1 -> On/1(Bass)
  FRComps/1 -> On/3(FRComps)
  FadeIn/1 -> On/4(FadeIn)
  Bypass/1(PremixOut) -> [PremixBypass]
  Bypass/2(FRMixerOut) -> [FRMBypass]
  Bypass/3(DgainsOut) -> [DgainsBypass]
  Bypass/4(PgainsOut) -> [PgainsBypass]
  [PremixBypass] -> Merge/2
  [FRMBypass] -> Merge1/2
  [DgainsBypass] -> Merge2/2
  [PgainsBypass] -> Merge3/2
  Selector4/1 -> FRMixerOut/1

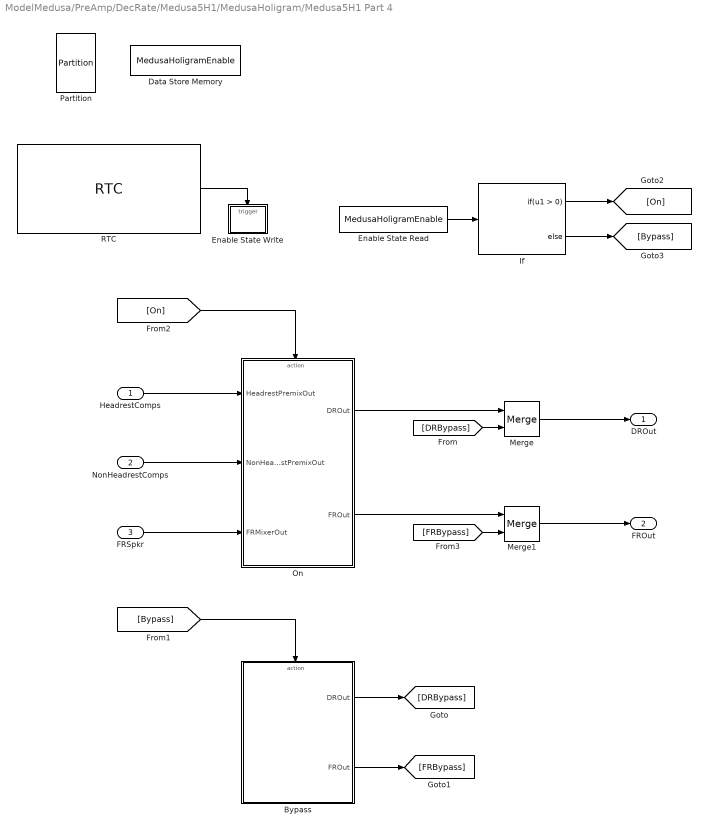
== system ModelMedusa/PreAmp/DecRate/Medusa5H1/MedusaHoligram/Medusa5H1 Part 4 ==
  HeadrestComps : Inport
  NonHeadrestComps : Inport  Port=2
  FRSpkr : Inport  Port=3
  Bypass : Subsystem
  Data Store Memory : DataStoreMemory  DataStoreName=MedusaHoligramEnable  ReadBeforeWriteMsg=warning  WriteAfterWriteMsg=warning  WriteAfterReadMsg=warning  InitialValue=1  ShowAdditionalParam=off  OutDataTypeStr=uint32
  Enable State Read : DataStoreRead  DataStoreName=MedusaHoligramEnable  IndexOptions=Index vector (dialog)  Indices=1  OutputSizes=1
  Enable State Write : Subsystem
  If : If
  Merge : Merge  InitialOutput=zeros(config.HoligramEQConfig.frameSize, config.numDRChan)
  Merge1 : Merge  InitialOutput=zeros(config.HoligramEQConfig.frameSizeFR, config.numMedusaOut)
  On : Subsystem
  Partition : FeaturePath/Partition  PartitionNumber=6  TriggerInit=[335 311 380 379]
      settings: SourceProductName=Bose Talaria
  RTC : RTC/RTC  REQ_Priority=RTC_Mask.NormalPriority  RequestAtInit=off  EnableRequest=on  REQElemType1=int32  REQElemWidth1=1  REQElemInitial1=[]  REQElemType2=uint32  REQElemWidth2=1  REQElemInitial2=[]  REQElemType3=uint32  REQElemWidth3=1  REQElemInitial3=[]  REQElemType4=uint32  REQElemWidth4=1  REQElemInitial4=[]  REQElemType5=uint32  REQElemWidth5=1  REQElemInitial5=[]  REQElemType6=uint32  REQElemWidth6=1  REQElemInitial6=[]  REQElemType7=uint32  REQElemWidth7=1  REQElemInitial7=[]  REQElemType8=uint32  REQElemWidth8=1  REQElemInitial8=[]  REQElemType9=uint32  REQElemWidth9=1  REQElemInitial9=[]  REQElemType10=uint32  REQElemWidth10=1  REQElemInitial10=[]  EnableResponse=on  EnableRSP_StatusIn=off  RSPElemType1=uint32  RSPElemWidth1=1  RSPElemType2=uint32  RSPElemWidth2=1  RSPElemType3=uint32  RSPElemWidth3=1  RSPElemType4=uint32  RSPElemWidth4=1  RSPElemType5=uint32  RSPElemWidth5=1  RSPElemType6=uint32  RSPElemWidth6=1  RSPElemType7=uint32  RSPElemWidth7=1  RSPElemType8=uint32  RSPElemWidth8=1  RSPElemType9=uint32  RSPElemWidth9=1  RSPElemType10=uint32  RSPElemWidth10=1  EnableNotification=off  EnableNTF_PrepTrig=off  NTFElemType1=uint32  NTFElemWidth1=1  NTFElemType2=uint32  NTFElemWidth2=1  NTFElemType3=uint32  NTFElemWidth3=1  NTFElemType4=uint32  NTFElemWidth4=1  NTFElemType5=uint32  NTFElemWidth5=1  NTFElemType6=uint32  NTFElemWidth6=1  NTFElemType7=uint32  NTFElemWidth7=1  NTFElemType8=uint32  NTFElemWidth8=1  NTFElemType9=uint32  NTFElemWidth9=1  NTFElemType10=uint32  NTFElemWidth10=1  MaskMessageName=HoligramDisable
      settings: SourceProductName=Bose Talaria
  DROut : Outport  VectorParamsAs1DForOutWhenUnconnected=off
  FROut : Outport  Port=2  VectorParamsAs1DForOutWhenUnconnected=off
  wires:
  Merge1/1 -> FROut/1
  On/2(FROut) -> Merge1/1
  RTC/1 -> Enable State Write/Trigger
  [On] -> On/Action
  Enable State Read/1 -> If/1
  If/2 -> [Bypass]
  If/1 -> [On]
  Merge/1 -> DROut/1
  On/1(DROut) -> Merge/1
  [Bypass] -> Bypass/Action
  FRSpkr/1 -> On/3(FRMixerOut)
  NonHeadrestComps/1 -> On/2(NonHeadrestPremixOut)
  HeadrestComps/1 -> On/1(HeadrestPremixOut)
  Bypass/1(DROut) -> [DRBypass]
  Bypass/2(FROut) -> [FRBypass]
  [DRBypass] -> Merge/2
  [FRBypass] -> Merge1/2

== system ModelMedusa/PreAmp/DecRate/Medusa5H1/MedusaHoligram/Medusa5H1 Part 5 ==
  DRIn : Inport
  FRIn : Inport  Port=2
  DR Speaker and HRComps Delay : MedusaDelays/MedusaTunableDelay  Config=Config.DeciRateSpeakerDelay
  FR Speaker Delay : MedusaDelays/MedusaTunableDelay  Config=Config.FullRateSpeakerDelay
  Partition : FeaturePath/Partition  PartitionNumber=7  TriggerInit=[1360 586 1405 654]
      settings: SourceProductName=Bose Talaria
  Speaker Delay Tune : Subsystem
  DROut : Outport  VectorParamsAs1DForOutWhenUnconnected=off
  FROut : Outport  Port=2  VectorParamsAs1DForOutWhenUnconnected=off
  wires:
  DR Speaker and HRComps Delay/1 -> DROut/1
  Speaker Delay Tune/2(FRSpeakerDelay) -> [FRSpeakerDelay]
  [DRSpeakerDelay] -> DR Speaker and HRComps Delay/2
  Speaker Delay Tune/1(DRSpeakerDelay) -> [DRSpeakerDelay]
  [FRSpeakerDelay] -> FR Speaker Delay/2
  FR Speaker Delay/1 -> FROut/1
  FRIn/1 -> FR Speaker Delay/1
  DRIn/1 -> DR Speaker and HRComps Delay/1

== system ModelMedusa/PreAmp/DecRate/Medusa5H1/MedusaHoligram/Medusa5H1 Part 1/CAE Treble Boost ==
  note: 1) Add Subsystem or Model blocks as valid variant choices.
      | 2) You cannot connect blocks at this level. At simulation, connectivity is automatically
      | determined, based on the active variant and port name matching.
  AudioIn : Inport
  Audio Passthrough : Subsystem  VariantControl=sys_defs.include_compressed_audio_enhancement == 0
  "CAE Treble Boost " : Subsystem  VariantControl=sys_defs.include_compressed_audio_enhancement == 1
  Out : Outport
  CAEEnable : Outport  Port=2

== system ModelMedusa/PreAmp/DecRate/Medusa5H1/MedusaHoligram/Medusa5H1 Part 1/Medusa Band Split Stereo ==
  LRhp : Inport
  Band Separation Delay : Delay  DelayLength=configStruct.band_separation_delay  InputProcessing=Columns as channels (frame based)
  Constant : Constant  Value=zeros(numInputs, 1)  OutDataTypeStr=uint32
  Downsample : DownSample  N=configStruct.D
  Image Rejection Filter : FIREven/FIR Even  variantSelect=Hexagon
      settings: SourceProductName=Bose Blocklib
  Image Rejection Filter Coeffs : Constant  Value=configStruct.fireven
  Interpolated Filter : Subsystem  AncestorBlock=Ifir/IFIR  mask(Interpolated FIR){coeffsFlip=configStruct.ifir, I=configStruct.D/2, numChannels=numInputs}
      mask prompts: coeffsFlip "Coefficients"; I "Interpolation Factor"; numChannels "Num inputs"
      mask help:
      | An interpolated FIR filter is an FIR filter with a sparse set of coefficients containing I-1 zeros between each point, where I is the interpolation factor.
      |
      | The block supports multiple channels, with each channel sharing the same set of filter coefficients. Users need to specify the non-zero coefficients, the interpolation factor and the number of channels.
      mask init:
      | % Flip the coeffs
      | [~, numCoeffSets] = size(coeffsFlip);
      | ind = 0:numCoeffSets-1;
      | coeffsFlip = flipud(coeffsFlip(:,ind+1));
      | 
      | % Cast decimation factor to int32
      | I = int32(I);
      settings: LibrarySourceBlock=Ifir/IFIR
  Reconstruction Filter : dspmlti4/FIR Interpolation  FilterSource=Dialog parameters  PrivateCoeffs=0  h=configStruct.upfir  L=configStruct.D  FilterObject=FINTERP  InputProcessing=Columns as channels (frame based)  framing=Enforce single-rate processing  outputBufInitCond=0  roundingMode=Floor  overflowMode=off  firstCoeffDataTypeStr=Inherit: Same word length as input  firstCoeffMin=[]  firstCoeffMax=[]  firstCoeffLastDataTypeStr=Inherit: Same word length as input  outputDataTypeStr=Inherit: Same as accumulator  outputMin=[]  outputMax=[]  outputLastDataTypeStr=Inherit: Same as accumulator
  Sum : Sum  Inputs=-+|
  LRbp : Outport  VectorParamsAs1DForOutWhenUnconnected=off
  LRtreble : Outport  Port=2  VectorParamsAs1DForOutWhenUnconnected=off
  wires:
  Constant/1 -> Image Rejection Filter/3
  Reconstruction Filter/1 -> Sum/1
  Interpolated Filter/1(AudioOut) -> Image Rejection Filter/1
  LRhp/1 -> Interpolated Filter/1(AudioIn), Band Separation Delay/1
  Image Rejection Filter Coeffs/1 -> Image Rejection Filter/2
  Image Rejection Filter/1 -> Downsample/1
  Sum/1 -> LRtreble/1
  Band Separation Delay/1 -> Sum/2
  Downsample/1 -> Reconstruction Filter/1, LRbp/1

== system ModelMedusa/PreAmp/DecRate/Medusa5H1/MedusaHoligram/Medusa5H1 Part 2/Alignment Delay ==
  LRhp : Inport
  Full-rate Alignment Delay Translation : MedusaDelays/MedusaFullRateAlignmentDelayTranslation  Config=Config.TrebleDelayTranslation
  Treble Delay : MedusaDelays/MedusaAlignmentDelay  Config=Config.TrebleDelay
  Tune Variable1 : TuneVar/TuneVar  TuneName=DeciRateNearWiggleFilterDelaySamples  SpecifyMaxSize=off  VariableDim=1 (Row)  MaxSize=[1 1]  TunabilityNumber=1  MinValue=[]  MaxValue=[]  TriggerInit=[-15 450 150 500]  MaskValue=Config.TrebleDelayTranslation.DefaultTuning.DeciRateNearWiggleDelay
      settings: SourceProductName=Bose Talaria
  Tune Variable4 : TuneVar/TuneVar  TuneName=DeciRateWiggleFilterDelaySamples  SpecifyMaxSize=off  VariableDim=1 (Row)  MaxSize=[1 1]  TunabilityNumber=1  MinValue=[]  MaxValue=[]  TriggerInit=[-15 385 150 435]  MaskValue=Config.TrebleDelayTranslation.DefaultTuning.DeciRateWiggleDelay
      settings: SourceProductName=Bose Talaria
  Tune Variable5 : TuneVar/TuneVar  TuneName=HoligramFilterAlignmentDelaySamples  SpecifyMaxSize=off  VariableDim=1 (Row)  MaxSize=[1 1]  TunabilityNumber=1  MinValue=[]  MaxValue=[]  TriggerInit=[-15 515 150 565]  MaskValue=Config.TrebleDelayTranslation.DefaultTuning.HoligramDelay
      settings: SourceProductName=Bose Talaria
  LRtreble : Outport
  wires:
  Tune Variable1/1 -> Full-rate Alignment Delay Translation/2  "DeciRateNearWiggleFilterDelaySamples"
  Tune Variable5/1 -> Full-rate Alignment Delay Translation/3  "HoligramFilterAlignmentDelaySamples"
  LRhp/1 -> Treble Delay/1
  Tune Variable4/1 -> Full-rate Alignment Delay Translation/1  "DeciRateWiggleFilterDelaySamples"
  Full-rate Alignment Delay Translation/1 -> [TrebleDelay]
  [TrebleDelay] -> Treble Delay/2
  Treble Delay/1 -> LRtreble/1  "LRtreble"

== system ModelMedusa/PreAmp/DecRate/Medusa5H1/MedusaHoligram/Medusa5H1 Part 3/Bypass ==
  Action Port : ActionPort  ActionPortLabel=else
  Constant : Constant  Value=zeros(config.HoligramEQConfig.frameSize, config.PremixConfig.NumPremixOut)  OutDataTypeStr=single
  Constant1 : Constant  Value=Config.DefaultFullRateMixerOutput  OutDataTypeStr=single
  Constant2 : Constant  Value=zeros(config.numVLSGains, 1)  OutDataTypeStr=single
  Constant3 : Constant  Value=zeros(config.numVLSGains, 1)  OutDataTypeStr=single
  PremixOut : Outport  VectorParamsAs1DForOutWhenUnconnected=off
  FRMixerOut : Outport  Port=2  VectorParamsAs1DForOutWhenUnconnected=off
  DgainsOut : Outport  Port=3  VectorParamsAs1DForOutWhenUnconnected=off
  PgainsOut : Outport  Port=4  VectorParamsAs1DForOutWhenUnconnected=off
  wires:
  Constant2/1 -> DgainsOut/1
  Constant3/1 -> PgainsOut/1
  Constant1/1 -> FRMixerOut/1
  Constant/1 -> PremixOut/1

== system ModelMedusa/PreAmp/DecRate/Medusa5H1/MedusaHoligram/Medusa5H1 Part 3/Enable State Write ==
  Trigger : TriggerPort  TriggerType=function-call  VariantControl=Variant  PortDimensions=1
  Constant : Constant  Value=0  OutDataTypeStr=uint32
  Data Store Write : DataStoreWrite  DataStoreName=MedusaPostUpmixEnable  IndexOptions=Index vector (dialog)  Indices=1  OutputSizes=1
  wires:
  Constant/1 -> Data Store Write/1

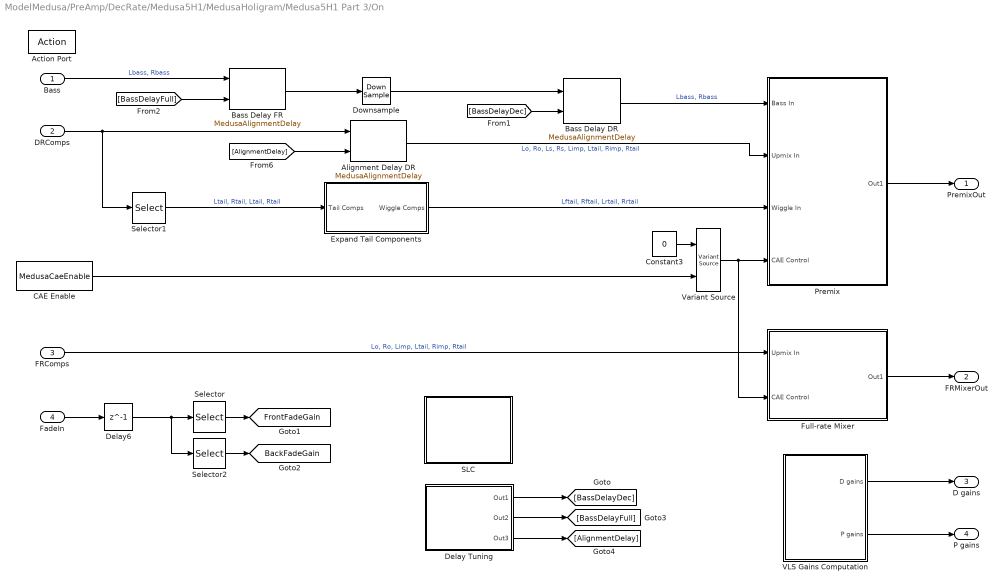
== system ModelMedusa/PreAmp/DecRate/Medusa5H1/MedusaHoligram/Medusa5H1 Part 3/On ==
  Bass : Inport  OutDataTypeStr=single
  DRComps : Inport  Port=2  OutDataTypeStr=single
  FRComps : Inport  Port=3  OutDataTypeStr=single
  FadeIn : Inport  Port=4  OutDataTypeStr=single
  Action Port : ActionPort  ActionPortLabel=if(u1 > 0)
  Alignment Delay DR : MedusaDelays/MedusaAlignmentDelay  Config=Config.MidrangeDelay
  Bass Delay DR : MedusaDelays/MedusaAlignmentDelay  Config=Config.DeciRateBassDelay
  Bass Delay FR : MedusaDelays/MedusaAlignmentDelay  Config=Config.FullRateBassDelay
  CAE Enable : MedusaCaeEnable/MedusaCaeEnable  Config=Config.PremixCaeEnable  MaskMessageName=PremixCAEEnable
  Constant3 : Constant  Value=0  OutDataTypeStr=int32  SampleTime=-1
  Delay Tuning : Subsystem
  Delay6 : Delay  DelayLength=1
  Downsample : DownSample  N=4
  Expand Tail Components : Subsystem  TreatAsAtomicUnit=on  RTWFileName=MedusaExpandTailComps
      settings: RTWSystemCode=Nonreusable function  RTWFileNameOpts=User specified  FunctionWithSeparateData=on
  Full-rate Mixer : Subsystem
  Premix : Subsystem
  SLC : Subsystem
  Selector : Selector  NumberOfDimensions=2  InputPortWidth=2  IndexOptions=Index vector (dialog),Index vector (dialog)  Indices=1,1  OutputSizes=1,1
  Selector1 : Selector  NumberOfDimensions=2  InputPortWidth=3  IndexOptions=Select all,Index vector (dialog)  Indices=[1 3],[6 8 6 8]  OutputSizes=1,1
  Selector2 : Selector  NumberOfDimensions=2  InputPortWidth=2  IndexOptions=Index vector (dialog),Index vector (dialog)  Indices=1,2  OutputSizes=1,1
  VLS Gains Computation : Subsystem
  Variant Source : VariantSource
  PremixOut : Outport  VectorParamsAs1DForOutWhenUnconnected=off
  FRMixerOut : Outport  Port=2  VectorParamsAs1DForOutWhenUnconnected=off
  D gains : Outport  Port=3
  P gains : Outport  Port=4
  tag scope: BackFadeGain=global, FrontFadeGain=global
  wires:
  Alignment Delay DR/1 -> Premix/2(Upmix In)  "Lo, Ro, Ls, Rs, Limp, Ltail, Rimp, Rtail"
  Variant Source/1 -> Full-rate Mixer/2(CAE Control), Premix/4(CAE Control)
  Constant3/1 -> Variant Source/1
  CAE Enable/1 -> Variant Source/2
  Full-rate Mixer/1(Out1) -> FRMixerOut/1
  FRComps/1 -> Full-rate Mixer/1(Upmix In)  "Lo, Ro, Limp, Ltail, Rimp, Rtail"
  Premix/1(Out1) -> PremixOut/1
  Expand Tail Components/1(Wiggle Comps) -> Premix/3(Wiggle In)  "Lftail, Rftail, Lrtail, Rrtail"
  Bass Delay DR/1 -> Premix/1(Bass In)  "Lbass, Rbass"
  VLS Gains Computation/2(P gains) -> P gains/1
  VLS Gains Computation/1(D gains) -> D gains/1
  Delay Tuning/3(Out3) -> [AlignmentDelay]
  Delay Tuning/2(Out2) -> [BassDelayFull]
  Delay Tuning/1(Out1) -> [BassDelayDec]
  DRComps/1 -> Alignment Delay DR/1, Selector1/1
  Downsample/1 -> Bass Delay DR/1
  [BassDelayDec] -> Bass Delay DR/2
  [AlignmentDelay] -> Alignment Delay DR/2
  [BassDelayFull] -> Bass Delay FR/2
  Bass/1 -> Bass Delay FR/1  "Lbass, Rbass"
  Selector1/1 -> Expand Tail Components/1(Tail Comps)  "Ltail, Rtail, Ltail, Rtail"
  Bass Delay FR/1 -> Downsample/1
  FadeIn/1 -> Delay6/1
  Selector2/1 -> [BackFadeGain]
  Delay6/1 -> Selector2/1, Selector/1
  Selector/1 -> [FrontFadeGain]

== system ModelMedusa/PreAmp/DecRate/Medusa5H1/MedusaHoligram/Medusa5H1 Part 4/Bypass ==
  Action Port : ActionPort  ActionPortLabel=else
  Constant : Constant  Value=zeros(config.HoligramEQConfig.frameSize, config.numDRChan)  OutDataTypeStr=single
  Constant1 : Constant  Value=zeros(config.HoligramEQConfig.frameSizeFR, config.numMedusaOut)  OutDataTypeStr=single
  DROut : Outport  VectorParamsAs1DForOutWhenUnconnected=off
  FROut : Outport  Port=2  VectorParamsAs1DForOutWhenUnconnected=off
  wires:
  Constant1/1 -> FROut/1
  Constant/1 -> DROut/1

== system ModelMedusa/PreAmp/DecRate/Medusa5H1/MedusaHoligram/Medusa5H1 Part 4/Enable State Write ==
  Trigger : TriggerPort  TriggerType=function-call  VariantControl=Variant  PortDimensions=1
  Constant : Constant  Value=0  OutDataTypeStr=uint32
  Data Store Write : DataStoreWrite  DataStoreName=MedusaHoligramEnable  IndexOptions=Index vector (dialog)  Indices=1  OutputSizes=1
  wires:
  Constant/1 -> Data Store Write/1
